simulink model "punto1"  (R2015a)
settings: Solver=ode45  StartTime=0.0  StopTime=100  RelTol=1e-3
libraries: simulink x4, cstblocks x2
settings Model: Creator=Jose Roldan  LastModifiedBy=Jose Roldan

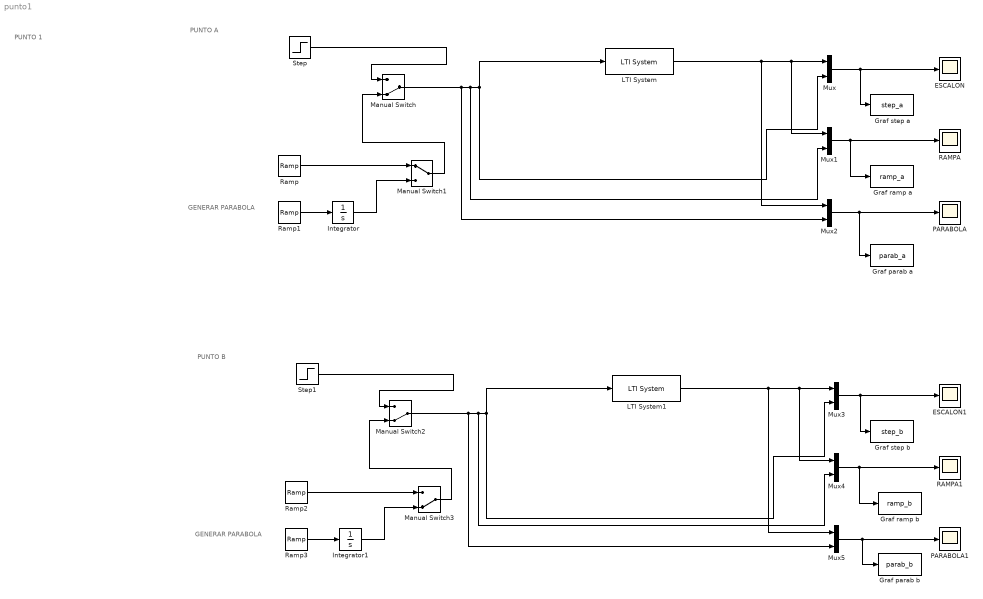
== system punto1 ==
  note: PUNTO 1
  note: PUNTO A
  note: GENERAR PARABOLA
  note: PUNTO B
  note: GENERAR PARABOLA
  ESCALON : Scope
  ESCALON1 : Scope
      settings: SaveName=ScopeData3
  Graf parab a : ToWorkspace  VariableName=parab_a  SaveFormat=Timeseries  SampleTime=-1
  Graf parab b : ToWorkspace  VariableName=parab_b  SaveFormat=Timeseries  SampleTime=-1
  "Graf ramp a " : ToWorkspace  VariableName=ramp_a  SaveFormat=Timeseries  SampleTime=-1
  Graf ramp b : ToWorkspace  VariableName=ramp_b  SaveFormat=Timeseries  SampleTime=-1
  Graf step a : ToWorkspace  VariableName=step_a  SaveFormat=Timeseries  SampleTime=-1
  "Graf step b " : ToWorkspace  VariableName=step_b  SaveFormat=Timeseries  SampleTime=-1
  Integrator : Integrator
  Integrator1 : Integrator
  LTI System : cstblocks/LTI System  sys=Ta  IC=[]
  LTI System1 : cstblocks/LTI System  sys=Tb  IC=[]
  Manual Switch : ManualSwitch  CurrentSetting=0
  Manual Switch1 : ManualSwitch
  Manual Switch2 : ManualSwitch  CurrentSetting=0
  Manual Switch3 : ManualSwitch  CurrentSetting=0
  Mux{,1..5} (6 alike) : Mux  Inputs=2
  PARABOLA : Scope
      settings: SaveName=ScopeData2
  PARABOLA1 : Scope
      settings: YMin=-10  YMax=60  SaveName=ScopeData4
  RAMPA : Scope
  RAMPA1 : Scope
      settings: SaveName=ScopeData5
  Ramp{,1..3} (4 alike) : simulink/Sources/Ramp  slope=1  start=0  X0=0
  Step : Step  SampleTime=0
  Step1 : Step  SampleTime=0
  wires:
  Step/1 -> Manual Switch/1
  Ramp1/1 -> Integrator/1
  Ramp/1 -> Manual Switch1/1
  Integrator/1 -> Manual Switch1/2
  Manual Switch1/1 -> Manual Switch/2
  LTI System/1 -> Mux1/1, Mux/1, Mux2/1
  Mux/1 -> Graf step a/1, ESCALON/1
  Mux1/1 -> "Graf ramp a "/1, RAMPA/1
  Mux2/1 -> Graf parab a/1, PARABOLA/1
  Manual Switch/1 -> Mux2/2, Mux1/2, LTI System/1, Mux/2
  Step1/1 -> Manual Switch2/1
  Ramp3/1 -> Integrator1/1
  Ramp2/1 -> Manual Switch3/1
  Integrator1/1 -> Manual Switch3/2
  Manual Switch3/1 -> Manual Switch2/2
  LTI System1/1 -> Mux5/1, Mux4/1, Mux3/1
  Mux3/1 -> "Graf step b "/1, ESCALON1/1
  Mux4/1 -> Graf ramp b/1, RAMPA1/1
  Mux5/1 -> Graf parab b/1, PARABOLA1/1
  Manual Switch2/1 -> Mux5/2, Mux4/2, LTI System1/1, Mux3/2
